simulink model "tSOFC"  (R2012b)
settings: Solver=ode45  StartTime=0.0  StopTime=10.0  RelTol=1e-3
settings Model: Creator=tlavelle  LastModifiedBy=tlavelle

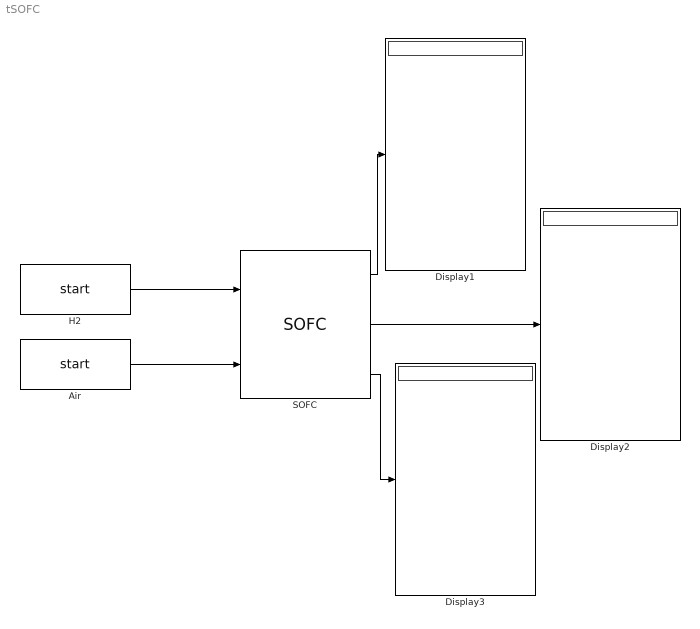
== system tSOFC ==
  Air : M-S-Function  FunctionName=start  Parameters=W,Tt,Pt,comp1,comp2,comp3,comp4,comp5,comp6,comp7,comp8,comp9,comp10  mask{W=1.0, Tt=1752, Pt=14.7, comp1=1, comp2=0, comp3=0, comp4=0, comp5=0, comp6=0, comp7=0, comp8=0, comp9=0, comp10=0}
      mask Display: color('blue'); port_label('output',1,'Flow Out')
  Display1 : Display
  Display2 : Display
  Display3 : Display
  H2 : M-S-Function  FunctionName=start  Parameters=W,Tt,Pt,comp1,comp2,comp3,comp4,comp5,comp6,comp7,comp8,comp9,comp10  mask{W=.0015, Tt=1752, Pt=14.7, comp1=0, comp2=.995, comp3=0, comp4=.005, comp5=0, comp6=0, comp7=0, comp8=0, comp9=0, comp10=0}
      mask Display: color('blue'); port_label('output',1,'Flow Out')
  SOFC : M-S-Function  FunctionName=SOFC  Parameters=AirStoich,Alpha,cellActiveArea,effIntercon,EidealStd,h_aOut,iDens,iDensExchange,iDensInternal,iDensLimit,LHVfuel,numCells,pAnode,pCathode,pctH2_lost,pctH2recyc_a,pctH2util,pctLossIntercon,pctO2_lost,resist,Temp,Z  mask{AirStoich=2.0, Alpha=1.54, cellActiveArea=400., effIntercon=1.0, EidealStd=1.18, h_aOut=0, iDens=826, iDensExchange=300., iDensInternal=2.0, iDensLimit=900., LHVfuel=0, numCells=237, pAnode=14.7, pCathode=14.7, pctH2_lost=1.0, pctH2recyc_a=0, pctH2util=.85, pctLossIntercon=.25, pctO2_lost=1.0, resist=.0003, Temp=1752, Z=2.0}
      mask Display:
      | color('blue'); port_label('input',1,'Flow Anode In')
      | color('blue'); port_label('input',2,'Flow Cathode In')
      | color('blue'); port_label('output',1,'Flow Anode Out')
      | color('blue'); port_label('output',2,'Flow Cathode Out')
      | color('blue'); port_label('output',3,'Output Data')
  wires:
  SOFC/1 -> Display1/1
  SOFC/2 -> Display2/1
  SOFC/3 -> Display3/1
  H2/1 -> SOFC/1
  Air/1 -> SOFC/2
